simulink model "humidity"  (R2020b)
settings: Solver=VariableStepAuto  StartTime=0.0  StopTime=10.0  RelTol=1e-3
settings Model: Creator=xinbo  LastModifiedBy=xinbo

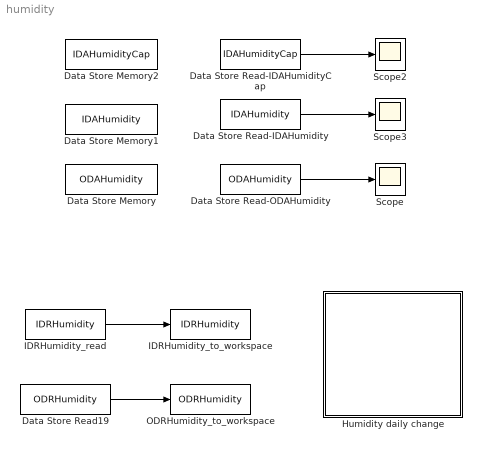
== system humidity ==
  Data Store Read-IDAHumidity : DataStoreRead  DataStoreName=IDAHumidity
  Data Store Read-IDAHumidityCap : DataStoreRead  DataStoreName=IDAHumidityCap
  Data Store Read-ODAHumidity : DataStoreRead  DataStoreName=ODAHumidity
  Data Store Read19 : DataStoreRead  DataStoreName=ODRHumidity
  Data Store Memory : DataStoreMemory  DataStoreName=ODAHumidity  ReadBeforeWriteMsg=warning  WriteAfterWriteMsg=warning  WriteAfterReadMsg=warning  ShowAdditionalParam=off
  Data Store Memory1 : DataStoreMemory  DataStoreName=IDAHumidity  ReadBeforeWriteMsg=warning  WriteAfterWriteMsg=warning  WriteAfterReadMsg=warning  ShowAdditionalParam=off
  Data Store Memory2 : DataStoreMemory  DataStoreName=IDAHumidityCap  ReadBeforeWriteMsg=warning  WriteAfterWriteMsg=warning  WriteAfterReadMsg=warning  ShowAdditionalParam=off
  Humidity daily change : Subsystem
      mask Display: image('$imagefile'); % Use "Edit Image" on toolstrip to change.
  IDRHumidity_read : DataStoreRead  DataStoreName=IDRHumidity
  IDRHumidity_to_workspace : ToWorkspace  VariableName=IDRHumidity  SampleTime=-1
      settings: Save2DSignal=2-D array (concatenate along first dimension)
  ODRHumidity_to_workspace : ToWorkspace  VariableName=ODRHumidity  SampleTime=-1
      settings: Save2DSignal=2-D array (concatenate along first dimension)
  Scope : Scope
  Scope2 : Scope
  Scope3 : Scope
  wires:
  Data Store Read19/1 -> ODRHumidity_to_workspace/1
  IDRHumidity_read/1 -> IDRHumidity_to_workspace/1
  Data Store Read-IDAHumidityCap/1 -> Scope2/1
  Data Store Read-IDAHumidity/1 -> Scope3/1
  Data Store Read-ODAHumidity/1 -> Scope/1

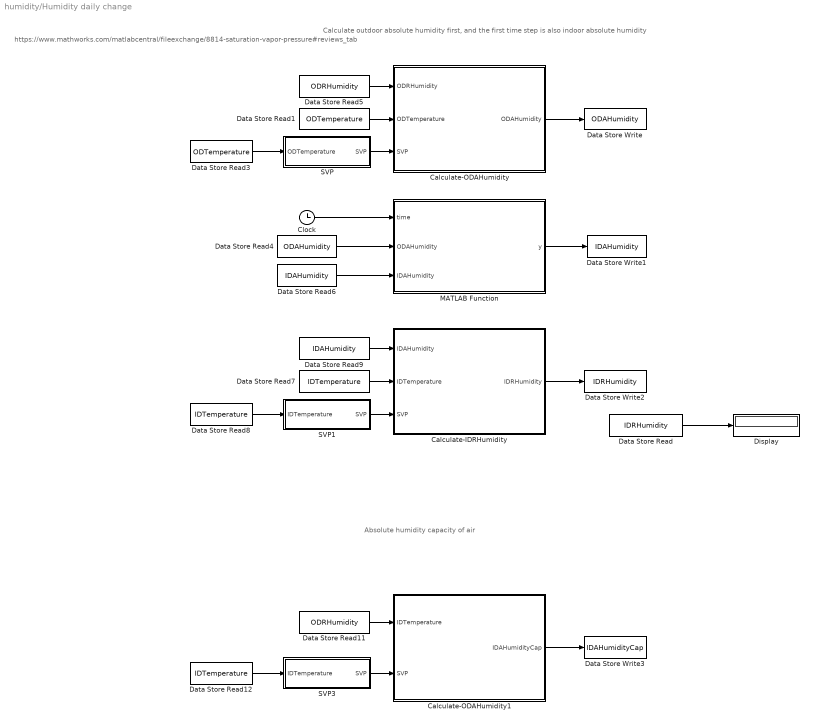
== system humidity/Humidity daily change ==
  note: Absolute humidity capacity of air
  note: https://www.mathworks.com/matlabcentral/fileexchange/8814-saturation-vapor-pressure#reviews_tab
  note: Calculate outdoor absolute humidity first, and the first time step is also indoor absolute humidity
  Calculate-IDRHumidity : MATLAB Function  TreatAsAtomicUnit=on
  Calculate-ODAHumidity : MATLAB Function  TreatAsAtomicUnit=on
  Calculate-ODAHumidity1 : MATLAB Function  TreatAsAtomicUnit=on
  Clock : Clock
  Data Store Read : DataStoreRead  DataStoreName=IDRHumidity
  Data Store Read1 : DataStoreRead  DataStoreName=ODTemperature
  Data Store Read11 : DataStoreRead  DataStoreName=ODRHumidity
  Data Store Read12 : DataStoreRead  DataStoreName=IDTemperature
  Data Store Read3 : DataStoreRead  DataStoreName=ODTemperature
  Data Store Read4 : DataStoreRead  DataStoreName=ODAHumidity
  Data Store Read5 : DataStoreRead  DataStoreName=ODRHumidity
  Data Store Read6 : DataStoreRead  DataStoreName=IDAHumidity
  Data Store Read7 : DataStoreRead  DataStoreName=IDTemperature
  Data Store Read8 : DataStoreRead  DataStoreName=IDTemperature
  Data Store Read9 : DataStoreRead  DataStoreName=IDAHumidity
  Data Store Write : DataStoreWrite  DataStoreName=ODAHumidity
  Data Store Write1 : DataStoreWrite  DataStoreName=IDAHumidity
  Data Store Write2 : DataStoreWrite  DataStoreName=IDRHumidity
  Data Store Write3 : DataStoreWrite  DataStoreName=IDAHumidityCap
  Display : Display
  MATLAB Function : MATLAB Function  TreatAsAtomicUnit=on
  SVP : MATLAB Function  TreatAsAtomicUnit=on
  SVP1 : MATLAB Function  TreatAsAtomicUnit=on
  SVP3 : MATLAB Function  TreatAsAtomicUnit=on
  wires:
  Data Store Read3/1 -> SVP/1(ODTemperature)
  Data Store Read5/1 -> Calculate-ODAHumidity/1(ODRHumidity)
  SVP/1(SVP) -> Calculate-ODAHumidity/3(SVP)
  Data Store Read1/1 -> Calculate-ODAHumidity/2(ODTemperature)
  Calculate-ODAHumidity/1(ODAHumidity) -> Data Store Write/1
  Clock/1 -> MATLAB Function/1(time)
  Data Store Read4/1 -> MATLAB Function/2(ODAHumidity)
  MATLAB Function/1(y) -> Data Store Write1/1
  Data Store Read6/1 -> MATLAB Function/3(IDAHumidity)
  Calculate-IDRHumidity/1(IDRHumidity) -> Data Store Write2/1
  SVP1/1(SVP) -> Calculate-IDRHumidity/3(SVP)
  Data Store Read9/1 -> Calculate-IDRHumidity/1(IDAHumidity)
  Data Store Read8/1 -> SVP1/1(IDTemperature)
  Data Store Read7/1 -> Calculate-IDRHumidity/2(IDTemperature)
  Data Store Read11/1 -> Calculate-ODAHumidity1/1(IDTemperature)
  Calculate-ODAHumidity1/1(IDAHumidityCap) -> Data Store Write3/1
  SVP3/1(SVP) -> Calculate-ODAHumidity1/2(SVP)
  Data Store Read12/1 -> SVP3/1(IDTemperature)
  Data Store Read/1 -> Display/1

== matlab function humidity/Humidity daily change/MATLAB Function ==
  data: time input; y output; ODAHumidity input; IDAHumidity input
function y = CalIDAHumidity(time, ODAHumidity, IDAHumidity)

if(time == 0)
    y = ODAHumidity;
else
    y = IDAHumidity;
end

== matlab function humidity/Humidity daily change/SVP ==
  data: SVP output; ODTemperature input
function SVP = svp(ODTemperature)

% [°C] = [K] - 273.15
% https://www.mathworks.com/matlabcentral/fileexchange/8814-saturation-vapor-pressure
% T = temperature on Kelvin scale
% SVP = saturation vapor pressure according to Goff & Gratch Equation (1946)
% SVP in Pascal

Ts = 373.15;    % standard temperature at steam point on Kelvin scale (Goff, 1965)
Ps = 101324.6;  % standard atmospheric pressure at steam point (Pascal)

T = ODTemperature + 273.15;
log10SVP = -7.90298*(Ts./T - 1) + 5.02808*log10(Ts./T) -1.3816e-7*(10.^(11.344*(1 - T./Ts)) - 1) + 8.1328e-3*(10.^(3.49149*(1 - Ts./T)) - 1) + log10(Ps);

SVP = 10.^(log10SVP);

== matlab function humidity/Humidity daily change/Calculate-IDRHumidity ==
  data: IDRHumidity output; IDAHumidity input; IDTemperature input; SVP input
function IDRHumidity = CalIDRHumidity(IDAHumidity, IDTemperature, SVP)

% https://www.mathworks.com/matlabcentral/fileexchange/8814-saturation-vapor-pressure

% ODTemperature in Celius
% [°C] = [K] - 273.15
% SVP = saturation vapor pressure according to Goff & Gratch Equation (1946)
% SVP in Pascal
% IDAHumidity is in kg/m3, absolute humidity


Rw = 461.5;
% J/(kg*K) Rw is specific gas constant for water vapor 
IDTemperature = IDTemperature + 273.15;

IDRHumidity = IDAHumidity * Rw * IDTemperature * 100 / SVP;

if (IDRHumidity > 100)
    IDRHumidity = 100;
end

== matlab function humidity/Humidity daily change/Calculate-ODAHumidity ==
  data: ODAHumidity output; ODRHumidity input; ODTemperature input; SVP input
function ODAHumidity = CalODAHumidity(ODRHumidity, ODTemperature, SVP)

% https://www.mathworks.com/matlabcentral/fileexchange/8814-saturation-vapor-pressure

% ODTemperature in Celius
% [°C] = [K] - 273.15
% SVP = saturation vapor pressure according to Goff & Gratch Equation (1946)
% SVP in Pascal
% ODAHumidity is in kg/m3

Rw = 461.5;
% J/(kg*K) Rw is specific gas constant for water vapor 
T = ODTemperature + 273.15;
ODAHumidity = ODRHumidity * SVP / (Rw * T * 100);

== matlab function humidity/Humidity daily change/SVP1 ==
  data: SVP output; IDTemperature input
function SVP = svp(IDTemperature)

% [°C] = [K] - 273.15
% https://www.mathworks.com/matlabcentral/fileexchange/8814-saturation-vapor-pressure
% T = temperature on Kelvin scale
% SVP = saturation vapor pressure according to Goff & Gratch Equation (1946)
% SVP in Pascal

Ts = 373.15;    % standard temperature at steam point on Kelvin scale (Goff, 1965)
Ps = 101324.6;  % standard atmospheric pressure at steam point (Pascal)

T = IDTemperature + 273.15;
log10SVP = -7.90298*(Ts./T - 1) + 5.02808*log10(Ts./T) -1.3816e-7*(10.^(11.344*(1 - T./Ts)) - 1) + 8.1328e-3*(10.^(3.49149*(1 - Ts./T)) - 1) + log10(Ps);

SVP = 10.^(log10SVP);

== matlab function humidity/Humidity daily change/Calculate-ODAHumidity1 ==
  data: IDAHumidityCap output; IDTemperature input; SVP input
function IDAHumidityCap = CalIDAHumidityCap(IDTemperature, SVP)

% https://www.mathworks.com/matlabcentral/fileexchange/8814-saturation-vapor-pressure

% ODTemperature in Celius
% [°C] = [K] - 273.15
% SVP = saturation vapor pressure according to Goff & Gratch Equation (1946)
% SVP in Pascal
% AHumidity is in kg/m3

Rw = 461.5;
% J/(kg*K) Rw is specific gas constant for water vapor 
T = IDTemperature + 273.15;
IDRHumidityCap = 100;
IDAHumidityCap = IDRHumidityCap * SVP / (Rw * T * 100);

== matlab function humidity/Humidity daily change/SVP3 ==
  data: SVP output; IDTemperature input
function SVP = svp(IDTemperature)

% [°C] = [K] - 273.15
% https://www.mathworks.com/matlabcentral/fileexchange/8814-saturation-vapor-pressure
% T = temperature on Kelvin scale
% SVP = saturation vapor pressure according to Goff & Gratch Equation (1946)
% SVP in Pascal

Ts = 373.15;    % standard temperature at steam point on Kelvin scale (Goff, 1965)
Ps = 101324.6;  % standard atmospheric pressure at steam point (Pascal)

T = IDTemperature + 273.15;
log10SVP = -7.90298*(Ts./T - 1) + 5.02808*log10(Ts./T) -1.3816e-7*(10.^(11.344*(1 - T./Ts)) - 1) + 8.1328e-3*(10.^(3.49149*(1 - Ts./T)) - 1) + log10(Ps);

SVP = 10.^(log10SVP);
